simulink model "hardware_design"  (R2024b)
settings: Solver=ode1  StartTime=0.0  StopTime=50  FixedStep=0.002  RelTol=1e-3  EnableMultiTasking=on
undefined symbols (not defined in the file or in its folder): HIL, qc_get_step_size
libraries: quarc_library x2, simulink x1
settings Model: SimulationMode=external  Creator=xli268  LastModifiedBy=yihui
settings SolverCC: AlgebraicLoopSolver=TrustRegion  PositivePriorityOrder=on
settings DataIOCC: ReturnWorkspaceOutputs=off
settings DebuggingCC: UnconnectedInputMsg=warning  UnconnectedOutputMsg=warning  UnconnectedLineMsg=warning  ArithmeticOperatorsInVariantConditions=warning
settings ModelReferenceCC: EnableRefExpFcnMdlSchedulingChecks=on
settings SFSimCC: SimUseLocalCustomCode=off  CustomCodeUndefinedFunction=UseInterfaceOnly
settings RTWCC: Description=QUARC Win64 Target  SystemTargetFile=quarc_win64.tlc  TemplateMakefile=quarc_default_tmf  RTWUseLocalCustomCode=off  GPUComputeCapability=3.5
settings STFCustomTargetCC: TargetPreCompLibLocation=C:\PROGRA~3\QUARC\lib\2018a\win64\release  TargetLangStandard=C99 (ISO)  ConcurrentExecutionCompliant=on  GRTInterface=on  SystemTargetFile=quarc_win64.tlc
settings GRTTargetCC: TargetPreCompLibLocation=C:\PROGRA~3\QUARC\lib\2018a\win64\release  ParMdlRefBuildCompliant=off  CompOptLevelCompliant=off  CombineOutputUpdateFcns=off  MatFileLogging=off  CPPClassGenCompliant=off  GRTInterface=on  UseToolchainInfoCompliant=off  ExtMode=on  ExtModeMexFile=quarc_comm

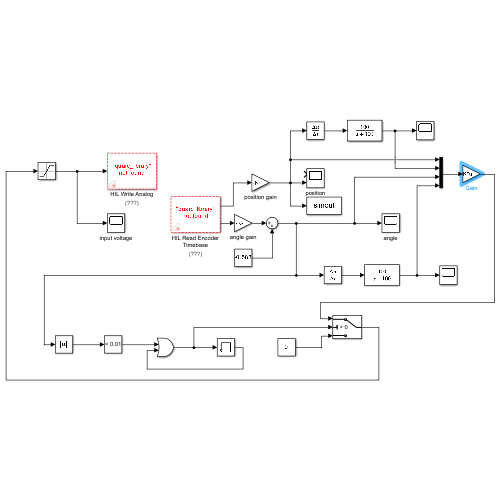
[thumbnail: Simulink's stored preview of the top-level diagram]
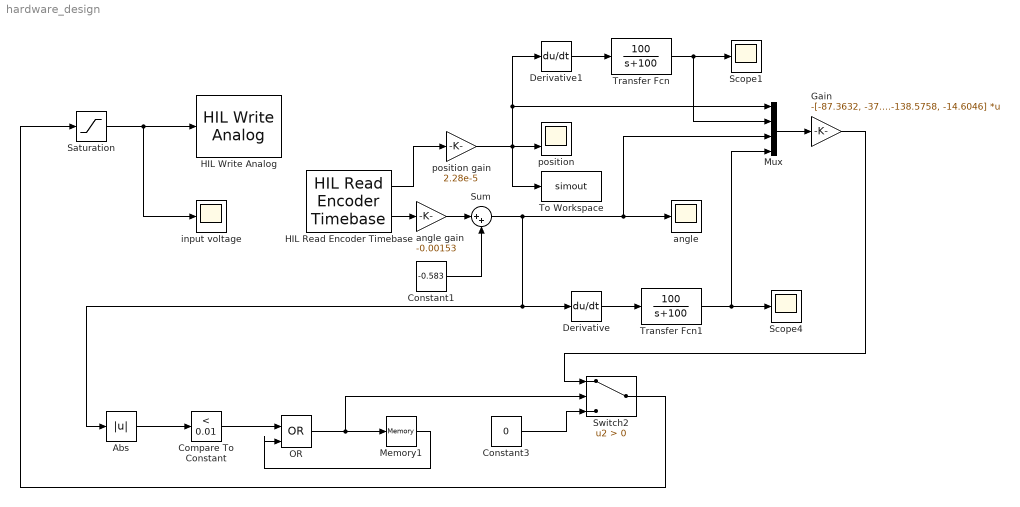
== system hardware_design ==
  Abs : Abs  SaturateOnIntegerOverflow=off
  Compare To Constant : simulink/Logic and Bit Operations/Compare To Constant  relop=<  const=0.01  OutDataTypeStr=boolean
  Constant1 : Constant  Value=-0.583
  Constant3 : Constant  Value=0
  Derivative : Derivative
  Derivative1 : Derivative
  Gain : Gain  Gain=-[-87.3632, -37.3740, -138.5758, -14.6046]  Multiplication=Matrix(K*u)
  HIL Read Encoder Timebase : quarc_library/Data Acquisition/Generic/Timebases/HIL Read Encoder Timebase  object_name=HIL-1  clock=0  channels=[0;1]  samples_in_buffer=max(ceil(1/qc_get_step_size), 1)  active=on  vector_output=off  data_type_mode=Inherit via back propagation  data_type=double
  HIL Write Analog : quarc_library/Data Acquisition/Generic/Immediate I//O/HIL Write Analog  object_name=HIL-1  channels=0  sample_time=-1  active=off  vector_input=off
  Memory1 : Memory
  Mux : Mux
  OR : Logic  Operator=OR  IconShape=distinctive  AllPortsSameDT=off  OutDataTypeStr=boolean
  Saturation : Saturate  UpperLimit=5  LowerLimit=-5
  Scope1 : Scope
  Scope4 : Scope
  Sum : Sum  Inputs=|++
  Switch2 : Switch  Criteria=u2 > Threshold  SaturateOnIntegerOverflow=off  InputSameDT=off
  To Workspace : ToWorkspace  VariableName=simout  SaveFormat=Structure With Time  SampleTime=-1
  Transfer Fcn : TransferFcn  Numerator=[100]  Denominator=[1 100]
  Transfer Fcn1 : TransferFcn  Numerator=[100]  Denominator=[1 100]
  angle : Scope
  "angle gain " : Gain  Gain=-0.00153
  input voltage : Scope
  position : Scope  NumInputPorts=2
  position gain : Gain  Gain=2.28e-5
  wires:
  Saturation/1 -> input voltage/1, HIL Write Analog/1
  position gain/1 -> To Workspace/1, Derivative1/1, Mux/1, position/2
  "angle gain "/1 -> Sum/1
  HIL Read Encoder Timebase/2 -> "angle gain "/1
  HIL Read Encoder Timebase/1 -> position gain/1
  Transfer Fcn1/1 -> Mux/4, Scope4/1
  Derivative1/1 -> Transfer Fcn/1
  Derivative/1 -> Transfer Fcn1/1
  Transfer Fcn/1 -> Mux/2, Scope1/1
  Constant1/1 -> Sum/2
  Sum/1 -> Derivative/1, Abs/1, Mux/3, angle/1
  Constant3/1 -> Switch2/3
  OR/1 -> Memory1/1, Switch2/2
  Memory1/1 -> OR/2
  Abs/1 -> Compare To Constant/1
  Mux/1 -> Gain/1
  Gain/1 -> Switch2/1
  Compare To Constant/1 -> OR/1
  Switch2/1 -> Saturation/1
